simulink model "QCar_CaptureScan"  (R2023a)
settings: Solver=ode1  StartTime=0.0  StopTime=inf  FixedStep=1/15  RelTol=1e-3  EnableMultiTasking=on
libraries: quarc_library x4, simulink x1
settings Model: SimulationMode=external  ExtModeTrigDuration=10000  Creator=PKaram  LastModifiedBy=SDRSADMIN
settings SolverCC: AlgebraicLoopSolver=TrustRegion  PositivePriorityOrder=on  AutoInsertRateTranBlk=on
settings DataIOCC: ReturnWorkspaceOutputs=off
settings DebuggingCC: ParameterPrecisionLossMsg=none  UnconnectedInputMsg=warning  UnconnectedOutputMsg=warning  UnconnectedLineMsg=warning  ArithmeticOperatorsInVariantConditions=warning
settings HardwareCC: ProdBitPerLong=64  ProdLargestAtomicFloat=None  ProdEndianess=Unspecified  ProdHWDeviceType=Generic->64-bit Embedded Processor (LP64)
settings ModelReferenceCC: EnableRefExpFcnMdlSchedulingChecks=on
settings SFSimCC: SimUseLocalCustomCode=off  CustomCodeUndefinedFunction=UseInterfaceOnly
settings RTWCC: Description=QUARC Linux Nvidia Target (QCar) Using Toolchain  SystemTargetFile=quarc_linux_nvidia.tlc  TemplateMakefile=quarc_linux_nvidia_tmf  RTWUseLocalCustomCode=off  Toolchain=QUARC linux_nvidia | gmake (64-bit Windows)  BuildConfiguration=Faster Runs  DLArmComputeVersion=19.05
settings CodeAppCC: StateflowObjectComments=on
settings STFCustomTargetCC: SystemTargetFile=quarc_linux_nvidia.tlc
settings GRTTargetCC: ParMdlRefBuildCompliant=off  CompOptLevelCompliant=off  CombineOutputUpdateFcns=off  MatFileLogging=off  CPPClassGenCompliant=off  GRTInterface=on  ExtMode=on  ExtModeMexFile=quarc_comm  ExtModeMexArgs='-w -d /home/nvidia/Documents -uri %u', 'tcpip://192.168.2.11:17001'
settings ConfigComp: CovMetricSettings=dswe

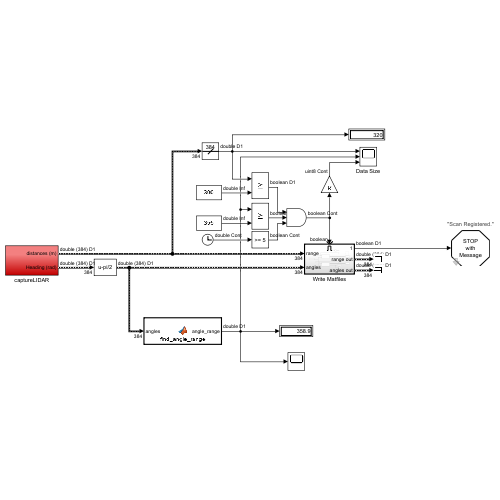
[thumbnail: Simulink's stored preview of the top-level diagram]
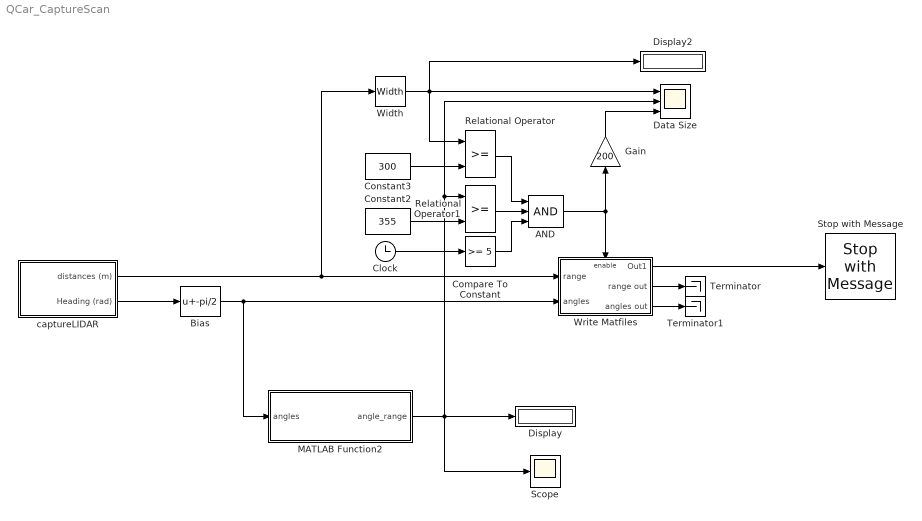
== system QCar_CaptureScan ==
  AND : Logic  Inputs=3  IconShape=distinctive  AllPortsSameDT=off  OutDataTypeStr=boolean
  Bias : Bias  Bias=-pi/2  SaturateOnIntegerOverflow=off
  Clock : Clock
  Compare To Constant : simulink/Logic and Bit Operations/Compare To Constant  relop=>=  const=5  OutDataTypeStr=boolean
  Constant2 : Constant  Value=355
  Constant3 : Constant  Value=300
  Data Size : Scope  NumInputPorts=3
  Display : Display
  Display2 : Display
  Gain : Gain  Gain=200
  MATLAB Function2 : MATLAB Function  TreatAsAtomicUnit=on
  Relational Operator : RelationalOperator  OutDataTypeStr=boolean  RndMeth=Simplest  InputSameDT=off
  Relational Operator1 : RelationalOperator  OutDataTypeStr=boolean  RndMeth=Simplest  InputSameDT=off
  Scope : Scope
  Stop with Message : quarc_library/Sinks/Error Handling/Stop with Message  message_type=Fixed error message  message_icon=Information  message=Scan Registered.
  Terminator : Terminator
  Terminator1 : Terminator
  Width : Width
  Write Matfiles : Subsystem  TreatAsAtomicUnit=on
  captureLIDAR : Subsystem
  wires:
  captureLIDAR/2(Heading (rad)) -> Bias/1
  captureLIDAR/1(distances (m)) -> Width/1, Write Matfiles/1(range)
  Width/1 -> Display2/1, Relational Operator/1, Data Size/1
  MATLAB Function2/1(angle_range) -> Data Size/2, Relational Operator1/1, Scope/1, Display/1
  Bias/1 -> MATLAB Function2/1(angles), Write Matfiles/2(angles)
  Constant3/1 -> Relational Operator/2
  Constant2/1 -> Relational Operator1/2
  Relational Operator/1 -> AND/1
  Relational Operator1/1 -> AND/2
  AND/1 -> Gain/1, Write Matfiles/Enable
  Gain/1 -> Data Size/3
  Write Matfiles/1(Out1) -> Stop with Message/1
  Write Matfiles/2(range out) -> Terminator/1
  Write Matfiles/3(angles out) -> Terminator1/1
  Clock/1 -> Compare To Constant/1
  Compare To Constant/1 -> AND/3

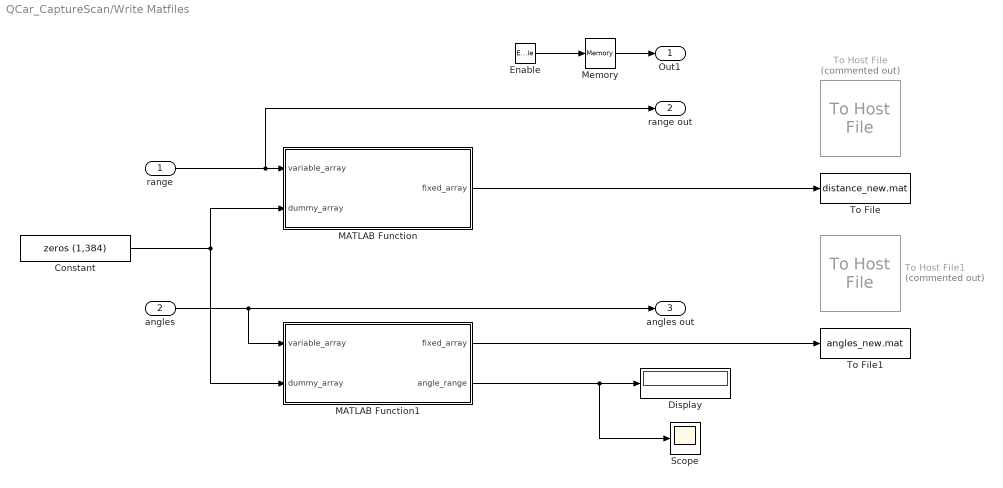
== system QCar_CaptureScan/Write Matfiles ==
  range : Inport
  angles : Inport  Port=2
  Enable : EnablePort  PropagateVarSize=During execution  ShowOutputPort=on
  Constant : Constant  Value=zeros (1,384)
  Display : Display
  MATLAB Function : MATLAB Function  TreatAsAtomicUnit=on
  MATLAB Function1 : MATLAB Function  TreatAsAtomicUnit=on
  Memory : Memory
  Scope : Scope
  To File : ToFile  Filename=distance_new.mat  MatrixName=distances
  To File1 : ToFile  Filename=angles_new.mat  MatrixName=angles
  To Host File : quarc_library/Sinks/To Host/To Host File  Commented=on  file_name=distance_new.mat  variable_name=distance_new  decimation=1  sample_time=-1  file_format=MAT-file v.4  options=No header or footer  append=off  final_file_name=distance_new.mat  bitrate=2000000
  To Host File1 : quarc_library/Sinks/To Host/To Host File  Commented=on  file_name=angles_new.mat  variable_name=angles_new  decimation=1  sample_time=-1  file_format=MAT-file v.4  options=No header or footer  append=off  final_file_name=angles_new.mat  bitrate=2000000
  Out1 : Outport
  range out : Outport  Port=2
  angles out : Outport  Port=3
  wires:
  range/1 -> range out/1, MATLAB Function/1(variable_array)
  MATLAB Function/1(fixed_array) -> To File/1
  angles/1 -> angles out/1, MATLAB Function1/1(variable_array)
  Constant/1 -> MATLAB Function/2(dummy_array), MATLAB Function1/2(dummy_array)
  MATLAB Function1/1(fixed_array) -> To File1/1
  MATLAB Function1/2(angle_range) -> Scope/1, Display/1
  Enable/1 -> Memory/1
  Memory/1 -> Out1/1

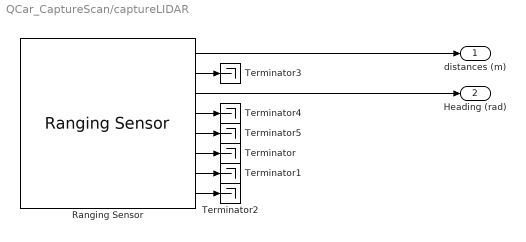
== system QCar_CaptureScan/captureLIDAR ==
  Ranging Sensor : quarc_library/Devices/Third-Party/Sensors/Ranging Sensor  sensor_type=RPLidar LIDAR  uri=serial-cpu://localhost:2?baud='115200',word='8',parity='none',stop='1',flow='none',dsr='on'  ranging_distance=Long  timing_budget=0.033  measurement_period=0.040  output_mode=Variable-size output  samples_per_revolution=384  max_distance=0.050  max_angle=5  sample_time=qc_get_step_size  show_versions=on  active=on
      settings: SourceProductName=QUARC Targets
  Terminator{,1..5} (6 alike) : Terminator
  distances (m) : Outport  VectorParamsAs1DForOutWhenUnconnected=off
  Heading (rad) : Outport  Port=2  VectorParamsAs1DForOutWhenUnconnected=off
  wires:
  Ranging Sensor/1 -> distances (m)/1
  Ranging Sensor/3 -> Heading (rad)/1
  Ranging Sensor/6 -> Terminator/1
  Ranging Sensor/7 -> Terminator1/1
  Ranging Sensor/8 -> Terminator2/1
  Ranging Sensor/2 -> Terminator3/1
  Ranging Sensor/4 -> Terminator4/1
  Ranging Sensor/5 -> Terminator5/1

== matlab function QCar_CaptureScan/MATLAB Function2 ==
  data: angles input; angle_range output
function angle_range = find_angle_range (angles)
angle_range = 0;
angle_range = max (angles) - min(angles);
angle_range = 180/pi*angle_range;

== matlab function QCar_CaptureScan/Write Matfiles/MATLAB Function1 ==
  data: variable_array input; fixed_array output; dummy_array input; angle_range output
function [fixed_array, angle_range] = make_fixed (variable_array, dummy_array)
fixed_array = dummy_array;
angle_range = 0;
for i = 1:length (variable_array)
    fixed_array(i) = variable_array (i);
end
% angle_range = variable_array(length (variable_array)) - variable_array(1);
angle_range = max (variable_array) - min(variable_array);
angle_range = 180/pi*angle_range;

== matlab function QCar_CaptureScan/Write Matfiles/MATLAB Function ==
  data: variable_array input; fixed_array output; dummy_array input
function fixed_array = make_fixed (variable_array, dummy_array)
fixed_array = dummy_array;
for i = 1:length (variable_array)
    fixed_array(i) = variable_array (i);
end
